simulink model "adaptiv_proj_6"  (R2015b)
settings: Solver=VariableStepAuto  StartTime=0.0  StopTime=10.0  RelTol=1e-3
values from neighbouring files (symbols this model uses):
  a0 = A(1)    [adaptiv_proj_61.m]
  a1 = A(2)    [adaptiv_proj_61.m]
  a2 = A(3)    [adaptiv_proj_61.m]
  am1 = 2*.9*sqrt(B)    [adaptiv_proj_61.m]
  am2 = B    (= 3056.76855895)    [adaptiv_proj_61.m]
  b0 = B    (= 3056.76855895)    [adaptiv_proj_61.m]
  bm = B    (= 3056.76855895)    [adaptiv_proj_61.m]
  g1 = g(1)    [adaptiv_proj_61.m]
  g2 = g(2)    [adaptiv_proj_61.m]
  g3 = g(3)    [adaptiv_proj_61.m]
settings Model: Creator=parviz  LastModifiedBy=parviz

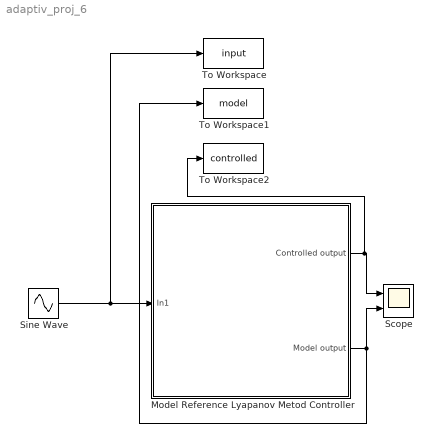
== system adaptiv_proj_6 ==
  Model Reference Lyapanov Metod Controller : Subsystem
  Scope : Scope  NumInputPorts=2
  Sine Wave : Sin  SampleTime=0
  To Workspace : ToWorkspace  VariableName=input  SaveFormat=Timeseries  SampleTime=-1
  To Workspace1 : ToWorkspace  VariableName=model  SaveFormat=Timeseries  SampleTime=-1
  To Workspace2 : ToWorkspace  VariableName=controlled  SaveFormat=Timeseries  SampleTime=-1
  wires:
  Sine Wave/1 -> To Workspace/1, Model Reference Lyapanov Metod Controller/1(In1)
  Model Reference Lyapanov Metod Controller/1(Controlled output) -> To Workspace2/1, Scope/1
  Model Reference Lyapanov Metod Controller/2(Model output) -> Scope/2, To Workspace1/1

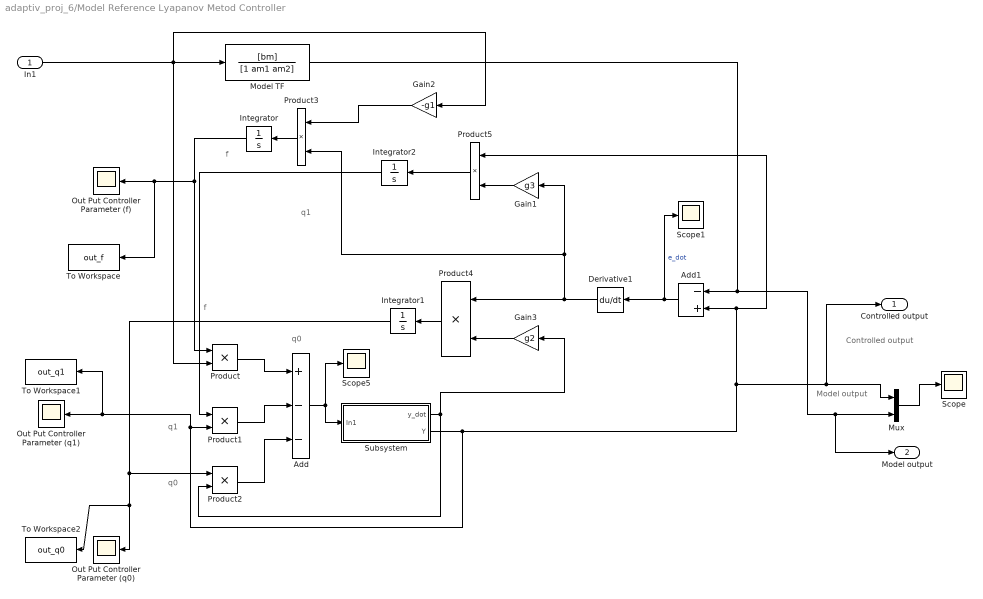
== system adaptiv_proj_6/Model Reference Lyapanov Metod Controller ==
  note: Controlled output
  note: Model output
  note: f
  note: f
  note: q0
  note: q1
  note: q0
  note: q1
  In1 : Inport
  Add : Sum  Inputs=+--
  Add1 : Sum  Inputs=-+
  Derivative1 : Derivative
  Gain1 : Gain  Gain=g3
  Gain2 : Gain  Gain=-g1
  Gain3 : Gain  Gain=g2
  Integrator : Integrator
  Integrator1 : Integrator
  Integrator2 : Integrator
  Model TF : TransferFcn  Numerator=[bm]  Denominator=[1 am1 am2]
  Mux : Mux  Inputs=2
  "Out Put Controller Parameter (f) " : Scope
  Out Put Controller Parameter (q0) : Scope
  Out Put Controller Parameter (q1) : Scope
  Product{,1..5} (6 alike) : Product
  Scope : Scope
  Scope1 : Scope
  Scope5 : Scope
  Subsystem : Subsystem
  To Workspace : ToWorkspace  VariableName=out_f  SaveFormat=Timeseries  SampleTime=-1
  To Workspace1 : ToWorkspace  VariableName=out_q1  SaveFormat=Timeseries  SampleTime=-1
  To Workspace2 : ToWorkspace  VariableName=out_q0  SaveFormat=Timeseries  SampleTime=-1
  Controlled output : Outport
  Model output : Outport  Port=2
  wires:
  Gain3/1 -> Product4/2
  Add/1 -> Scope5/1, Subsystem/1(In1)
  Model TF/1 -> Model output/1, Mux/2, Add1/1
  Subsystem/1(y_dot) -> Gain3/1, Product2/2
  Integrator/1 -> Product/1, "Out Put Controller Parameter (f) "/1, To Workspace/1
  Product2/1 -> Add/3
  Mux/1 -> Scope/1
  Add1/1 -> Derivative1/1, Scope1/1  "e_dot"
  Derivative1/1 -> Product4/1, Product3/2, Gain1/1
  Gain2/1 -> Product3/1
  Product3/1 -> Integrator/1
  In1/1 -> Product/2, Gain2/1, Model TF/1
  Product/1 -> Add/1
  Integrator2/1 -> Product1/1
  Product1/1 -> Add/2
  Product4/1 -> Integrator1/1
  Product5/1 -> Integrator2/1
  Gain1/1 -> Product5/2
  Subsystem/2("Y ") -> Product1/2, To Workspace1/1, Out Put Controller Parameter (q1)/1, Product5/1, Add1/2, Controlled output/1, Mux/1
  Integrator1/1 -> To Workspace2/1, Out Put Controller Parameter (q0)/1, Product2/1

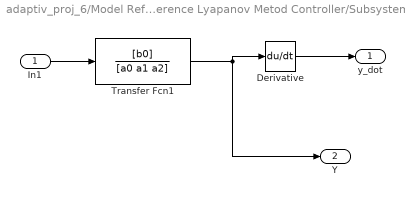
== system adaptiv_proj_6/Model Reference Lyapanov Metod Controller/Subsystem ==
  In1 : Inport
  Derivative : Derivative
  Transfer Fcn1 : TransferFcn  Numerator=[b0]  Denominator=[a0 a1 a2]
  y_dot : Outport
  "Y " : Outport  Port=2
  wires:
  Derivative/1 -> y_dot/1
  Transfer Fcn1/1 -> Derivative/1, "Y "/1
  In1/1 -> Transfer Fcn1/1
